simulink model "Demo_1"  (R2024b)
settings: Solver=FixedStepAuto  StartTime=0.0  StopTime=70.0  FixedStep=0.01  RelTol=1e-3
libraries: cstblocks x2, simulink x1, SignalEditorBlockLib x1
settings Model: Creator=Marcin  LastModifiedBy=Marcin

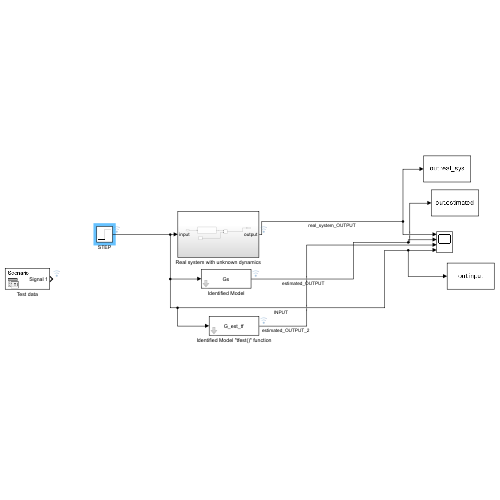
[thumbnail: Simulink's stored preview of the top-level diagram]
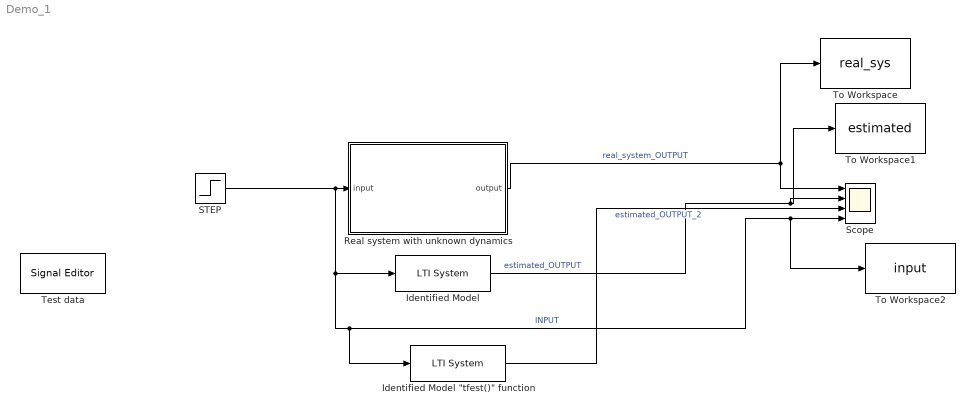
== system Demo_1 ==
  Identified Model : cstblocks/LTI System  sys=Gs  IC=[]  PadeOrder=0
  "Identified Model \"tfest()\" function" : cstblocks/LTI System  sys=G_est_tf  IC=[]  PadeOrder=0
  Real system with unknown dynamics : Subsystem
  STEP : Step  Time=10  SampleTime=0
  Scope : Scope  NumInputPorts=4
  Test data : SignalEditorBlockLib/Signal Editor  FileName=test_excitation_signal.mat  ActiveScenario=Scenario  ActiveSignal=Signal 1  IsBus=off  OutputBusObjectStr=Bus: BusObject  SampleTime=0  Interpolate=off  ZeroCross=off  OutputAfterFinalValue=Setting to zero  Unit=inherit  PreserveSignalName=on  ApplySigPropsToAllScenarios=on  ApplySigPropsToAllSignals=off
  To Workspace : ToWorkspace  VariableName=real_sys  SaveFormat=Timeseries  SampleTime=-1
  To Workspace1 : ToWorkspace  VariableName=estimated  SaveFormat=Timeseries  SampleTime=-1
  To Workspace2 : ToWorkspace  VariableName=input  SaveFormat=Timeseries  SampleTime=-1
  wires:
  Real system with unknown dynamics/1(output) -> Scope/1, To Workspace/1  "real_system_OUTPUT"
  Identified Model/1 -> To Workspace1/1, Scope/2  "estimated_OUTPUT"
  STEP/1 -> Identified Model/1, "Identified Model \"tfest()\" function"/1, To Workspace2/1, Scope/4, Real system with unknown dynamics/1(input)  "INPUT"
  "Identified Model \"tfest()\" function"/1 -> Scope/3  "estimated_OUTPUT_2"

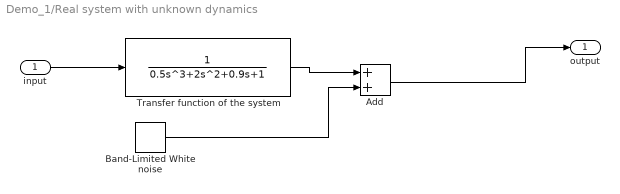
== system Demo_1/Real system with unknown dynamics ==
  input : Inport
  Add : Sum
  Band-Limited White noise : simulink/Sources/Band-Limited White Noise  Cov=[0.00006]  Ts=0.05  seed=[23331]
  Transfer function of the system : TransferFcn  Denominator=[0.5 2 0.9 1]
  output : Outport
  wires:
  Transfer function of the system/1 -> Add/1
  Band-Limited White noise/1 -> Add/2
  Add/1 -> output/1
  input/1 -> Transfer function of the system/1
